simulink model "testBFS"  (Simulink 7.4)
settings: Solver=ode45  StartTime=0.0  StopTime=10.0  MaxStep=0.01  RelTol=1e-3
undefined symbols (not defined in the file or in its folder): sparse, x1, x2
libraries: BLOM_Lib x11
settings Model: Creator=JJK  LastModifiedBy=JJK
settings DebuggingCC: SolverPrmCheckMsg=none

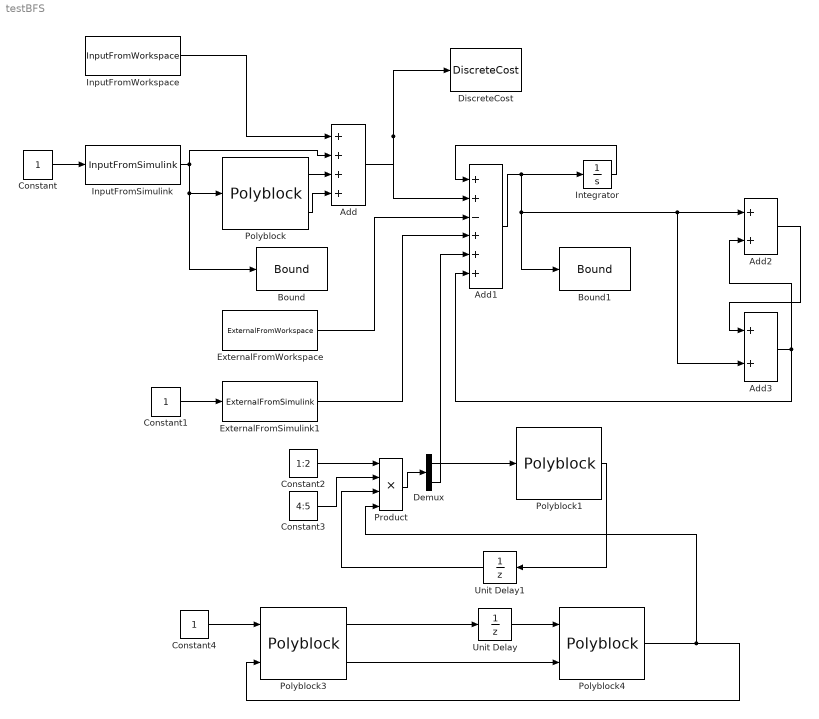
== system testBFS ==
  Add : Sum  Inputs=++++
  Add1 : Sum  Inputs=++-+++
  Add2 : Sum
  Add3 : Sum
  Bound : BLOM_Lib/Bound  SystemSampleTime=-1  ub=inf  lb=-inf  initial_step=on  final_step=on  intermediate_step=on
  Bound1 : BLOM_Lib/Bound  SystemSampleTime=-1  ub=inf  lb=-inf  initial_step=on  final_step=on  intermediate_step=on
  Constant : Constant
  Constant1 : Constant
  Constant2 : Constant  Value=1:2
  Constant3 : Constant  Value=4:5
  Constant4 : Constant
  Demux : Demux  Outputs=2
  DiscreteCost : BLOM_Lib/DiscreteCost  SystemSampleTime=-1  initial_step=on  final_step=on  intermediate_step=on
  ExternalFromSimulink1 : BLOM_Lib/ExternalFromSimulink  SystemSampleTime=-1  interpType=Zero-Order Hold
  ExternalFromWorkspace : BLOM_Lib/ExternalFromWorkspace  SystemSampleTime=-1  simin=simin  interpType=Zero-Order Hold
  InputFromSimulink : BLOM_Lib/InputFromSimulink  SystemSampleTime=-1  interpType=Zero-Order Hold
  InputFromWorkspace : BLOM_Lib/InputFromWorkspace  SystemSampleTime=-1  simin=simin  interpType=Zero-Order Hold
  Integrator : Integrator
  Polyblock : BLOM_Lib/Polyblock  SystemSampleTime=-1  P=sparse([1 1 0; 3 1 0])  K=sparse([1 0.8; 1 1])  inputs=x1,x2  inputScalar=on  outputScalar=on
  Polyblock1 : BLOM_Lib/Polyblock  SystemSampleTime=-1  P=sparse([1 1; 3 1])  K=sparse([1 0.8])  inputs=x1,x2  inputScalar=on  outputScalar=on
  Polyblock3 : BLOM_Lib/Polyblock  SystemSampleTime=-1  P=sparse([1 0 1 0; 3 0 1 0])  K=sparse([1 0.8; 1 1])  inputs=x1,x2  inputScalar=on  outputScalar=on
  Polyblock4 : BLOM_Lib/Polyblock  SystemSampleTime=-1  P=sparse([1 1 0; 3 1 0])  K=sparse([1 0.8])  inputs=x1,x2  inputScalar=on  outputScalar=on
  Product : Product  Inputs=4  RndMeth=Zero
  Unit Delay : UnitDelay  SampleTime=-1
  Unit Delay1 : UnitDelay  SampleTime=-1
  wires:
  Constant/1 -> InputFromSimulink/1
  InputFromWorkspace/1 -> Add/1
  Add/1 -> DiscreteCost/1, Add1/2
  Integrator/1 -> Add1/1
  Add1/1 -> Integrator/1, Bound1/1, Add2/1, Add3/2
  ExternalFromWorkspace/1 -> Add1/3
  ExternalFromSimulink1/1 -> Add1/4
  Constant1/1 -> ExternalFromSimulink1/1
  Polyblock/1 -> Add/3
  InputFromSimulink/1 -> Add/2, Bound/1, Polyblock/1
  Constant2/1 -> Product/1
  Constant3/1 -> Product/2
  Product/1 -> Demux/1
  Demux/1 -> Polyblock1/1
  Polyblock1/1 -> Unit Delay1/1
  Demux/2 -> Add1/5
  Add3/1 -> Add2/2, Add1/6
  Add2/1 -> Add3/1
  Unit Delay/1 -> Polyblock4/1
  Polyblock3/1 -> Unit Delay/1
  Unit Delay1/1 -> Product/3
  Polyblock3/2 -> Polyblock4/2
  Polyblock4/1 -> Product/4, Polyblock3/2
  Constant4/1 -> Polyblock3/1
  Polyblock/2 -> Add/4
